simulink subsystem "Communication"  (R2022b)
settings: Solver=VariableStepAuto  StartTime=0.0  StopTime=10.0  RelTol=1e-3
values from neighbouring files (symbols this model uses):
  PWMclock = 100000000    [SimDefaultParam.mat]
undefined symbols (not defined in the file or in its folder): Fi, ODR, samplerate_serial, samplerate_udp, Wi
libraries: arduinowifilib x3, svdutilitieslib x2, simulink x1, arduinosensorlib x1
settings Model: Creator=ReiterTo  LastModifiedBy=ReiterTo

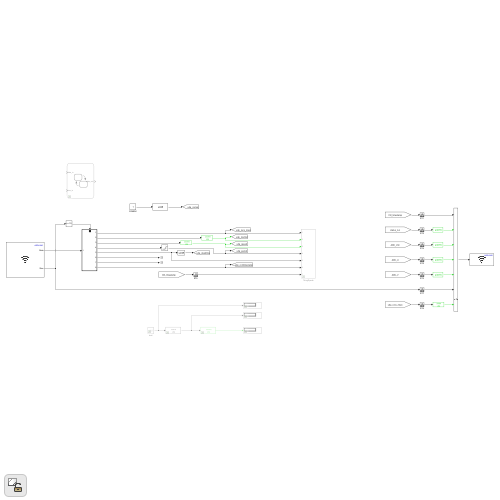
[thumbnail: Simulink's stored preview of the top-level diagram]
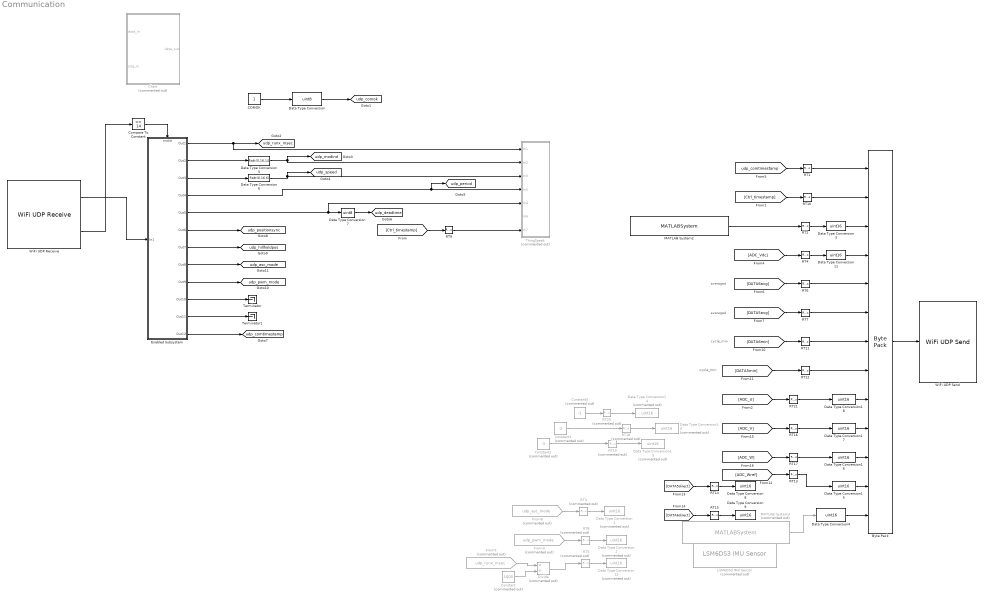
== system Communication ==
  note: averaged
  note: averaged
  note: cycle_min
  note: cycle_min
  Byte Pack : svdutilitieslib/Byte Pack  maskPackedDataType=uint16  datatypes={'uint32','uint32','uint16','uint16','uint16','uint16','uint16','uint16','uint16','uint16','uint16','uint16','uint16'}  byteAlign=2  blockPlatform=arduinoert
  COMOK : Constant  SampleTime=samplerate_serial
  Chart : Stateflow chart  Commented=on  TreatAsAtomicUnit=on
  Compare To Constant : simulink/Logic and Bit Operations/Compare To Constant  relop===  const=14  OutDataTypeStr=uint8
  Constant : Constant  Commented=on  Value=1000  OutDataTypeStr=uint16  SampleTime=samplerate_udp
  Constant1 : Constant  Commented=on  Value=-2  OutDataTypeStr=int16  SampleTime=samplerate_udp
  Constant2 : Constant  Commented=on  Value=-3  OutDataTypeStr=int16  SampleTime=samplerate_udp
  Constant3 : Constant  Commented=on  Value=-1  OutDataTypeStr=int16  SampleTime=samplerate_udp
  Data Type Conversion : DataTypeConversion  OutDataTypeStr=uint8  RndMeth=Simplest  SaturateOnIntegerOverflow=off
  Data Type Conversion1 : DataTypeConversion  Commented=on  OutDataTypeStr=uint16  RndMeth=Simplest  SaturateOnIntegerOverflow=off
  Data Type Conversion10 : DataTypeConversion  Commented=on  OutDataTypeStr=uint16  ConvertRealWorld=Stored Integer (SI)  RndMeth=Simplest  SaturateOnIntegerOverflow=off
  Data Type Conversion{3..4,8..9,11} (5 alike) : DataTypeConversion  OutDataTypeStr=uint16  RndMeth=Simplest  SaturateOnIntegerOverflow=off
  Data Type Conversion12 : DataTypeConversion  Commented=on  OutDataTypeStr=uint16  RndMeth=Simplest  SaturateOnIntegerOverflow=off
  Data Type Conversion13 : DataTypeConversion  Commented=on  OutDataTypeStr=uint16  ConvertRealWorld=Stored Integer (SI)  RndMeth=Simplest  SaturateOnIntegerOverflow=off
  Data Type Conversion14 : DataTypeConversion  Commented=on  OutDataTypeStr=uint16  ConvertRealWorld=Stored Integer (SI)  RndMeth=Simplest  SaturateOnIntegerOverflow=off
  Data Type Conversion{15..18} (4 alike) : DataTypeConversion  OutDataTypeStr=uint16  ConvertRealWorld=Stored Integer (SI)  RndMeth=Simplest  SaturateOnIntegerOverflow=off
  Data Type Conversion2 : DataTypeConversion  Commented=on  OutDataTypeStr=uint16  RndMeth=Simplest  SaturateOnIntegerOverflow=off
  Data Type Conversion5 : DataTypeConversion  OutDataTypeStr=fixdt(0,16,14)  ConvertRealWorld=Stored Integer (SI)  RndMeth=Simplest  SaturateOnIntegerOverflow=off  LockScale=on
  Data Type Conversion6 : DataTypeConversion  OutDataTypeStr=fixdt(0,16,6)  ConvertRealWorld=Stored Integer (SI)  RndMeth=Simplest  SaturateOnIntegerOverflow=off  LockScale=on
  Data Type Conversion7 : DataTypeConversion  OutDataTypeStr=uint8  RndMeth=Simplest  SaturateOnIntegerOverflow=off
  Divide : Product  Commented=on  Inputs=*/  OutDataTypeStr=uint32  RndMeth=Simplest
  Enabled Subsystem : Subsystem  TreatAsAtomicUnit=on
  From3 : From  Commented=on  GotoTag=udp_pwm_mode  TagVisibility=global
  From8 : From  Commented=on  GotoTag=udp_asc_mode  TagVisibility=global
  From9 : From  Commented=on  GotoTag=udp_runx_msec  TagVisibility=global
  LSM6DS3 IMU Sensor : arduinosensorlib/LSM6DS3 IMU Sensor  Commented=on  I2CAddress=0x6A  IsActiveAcceleration=off  IsActiveAngularRate=off  IsActiveTemperature=on  IsActiveStatus=off  IsActiveTimeStamp=off  spf=1  SampleTime=1  QueueSizeFactor=1  AccelerometerRange=+/- 2g  AccelerometerODR=12.5 Hz  SelectAnalogBW=off  AccelLPF1BW=400 Hz  AccelSelectCompositeFilter=No filter  AccelLPF2BW=ODR/50  AccelHPFBW=ODR/100  GyroscopeRange=250 dps  GyroscopeODR=12.5 Hz  SelectGyroscopeHPF=off  GyroHPFBW=0.0081 Hz
  MATLAB System2 : MATLABSystem  System=invPWM_Status
      mask Type: invPWM_Status
      mask Display:
      | disp('Inverter PWM Arduino Nano 33 IoT');
      | port_label('output',1,'pwm_run');
  MATLAB System3 : MATLABSystem  Commented=on  System=invSPI
      mask Type: invSPI
      mask Display:
      | disp('Inverter SPI Arduino Nano 33 IoT');
      | port_label('output',1,'DCL_RAW');
  RT{1..2,4,6..7,10..17,21} (14 alike) : RateTransition  Integrity=off  Deterministic=off  OutPortSampleTime=samplerate_udp
  RT{3,5,8,18..20} (6 alike) : RateTransition  Commented=on  Integrity=off  Deterministic=off  OutPortSampleTime=samplerate_udp
  RT9 : RateTransition  Integrity=off  Deterministic=off  OutPortSampleTime=samplerate_serial
  Terminator : Terminator
  Terminator1 : Terminator
  ThingSpeak : Subsystem  Commented=on
  WiFi UDP Receive : arduinowifilib/WiFi UDP Receive  localport=50000  DataType=uint16  DataLength=14  SampleTime_=samplerate_udp  wifiUDPIndex=0  blockPlatform=ARDUINO  isARMArch=true
  WiFi UDP Send : arduinowifilib/WiFi UDP Send  remoteIPOctetString=255.255.255.255  remoteport=60000  localport=50000  remoteipoctet1=255  remoteipoctet2=255  remoteipoctet3=255  remoteipoctet4=255  wifiUDPIndex=0  blockPlatform=ARDUINO  isARMArch=true
  tag scope: udp_asc_mode=global, udp_comok=global, udp_comtimestamp=global, udp_deadtime=global, udp_hillholdpos=global, udp_modind=global, udp_period=global, udp_positionsync=global, udp_pwm_mode=global, udp_runx_msec=global, udp_speed=global
  wires:
  Data Type Conversion/1 -> [udp_comok]
  [Ctrl_timestamp] -> RT9/1
  COMOK/1 -> Data Type Conversion/1
  RT2/1 -> Data Type Conversion3/1
  MATLAB System2/1 -> RT2/1
  RT1/1 -> Byte Pack/1
  Byte Pack/1 -> WiFi UDP Send/1
  Data Type Conversion6/1 -> ThingSpeak/3(In3), [udp_speed]
  Data Type Conversion7/1 -> [udp_deadtime]
  Enabled Subsystem/4(Out4) -> [udp_period], ThingSpeak/4(In5)
  [ADC_Vdc] -> RT4/1
  RT4/1 -> Data Type Conversion11/1
  From9/1 -> Divide/1
  RT5/1 -> Data Type Conversion12/1
  RT9/1 -> ThingSpeak/7(In7)
  RT3/1 -> Data Type Conversion1/1
  Data Type Conversion5/1 -> [udp_modind], ThingSpeak/2(In2)
  Enabled Subsystem/1(Out1) -> ThingSpeak/1(In1), [udp_runx_msec]
  Enabled Subsystem/5(Out5) -> Data Type Conversion7/1, ThingSpeak/5(In4)
  WiFi UDP Receive/1 -> Enabled Subsystem/1(In1)
  Enabled Subsystem/2(Out2) -> Data Type Conversion5/1
  Enabled Subsystem/3(Out3) -> Data Type Conversion6/1
  Enabled Subsystem/6(Out6) -> [udp_positionsync]
  Enabled Subsystem/7(Out7) -> [udp_hillholdpos]
  [DATA5avg] -> RT7/1
  [DATA6avg] -> RT6/1
  RT8/1 -> Data Type Conversion2/1
  WiFi UDP Receive/2 -> Compare To Constant/1
  Compare To Constant/1 -> Enabled Subsystem/Enable
  From3/1 -> RT8/1
  From8/1 -> RT3/1
  Enabled Subsystem/8(Out8) -> [udp_asc_mode]
  Enabled Subsystem/9(Out9) -> [udp_pwm_mode]
  Enabled Subsystem/10(Out10) -> Terminator/1
  Enabled Subsystem/11(Out11) -> Terminator1/1
  Divide/1 -> RT5/1
  Constant/1 -> Divide/2
  Enabled Subsystem/12(Out12) -> [udp_comtimestamp]
  [udp_comtimestamp] -> RT1/1
  [Ctrl_timestamp] -> RT10/1
  RT10/1 -> Byte Pack/2
  [DATA6min] -> RT11/1
  [DATA5min] -> RT12/1
  Data Type Conversion3/1 -> Byte Pack/3
  Data Type Conversion11/1 -> Byte Pack/4
  RT6/1 -> Byte Pack/5
  RT7/1 -> Byte Pack/6
  RT11/1 -> Byte Pack/7
  RT12/1 -> Byte Pack/8
  [DATA5direct] -> RT14/1
  RT14/1 -> Data Type Conversion8/1
  RT15/1 -> Data Type Conversion9/1
  [DATA6direct] -> RT15/1
  [ADC_V] -> RT16/1
  [ADC_W] -> RT17/1
  RT18/1 -> Data Type Conversion10/1
  [ADC_Wref] -> RT13/1
  RT13/1 -> Data Type Conversion15/1
  Data Type Conversion4/1 -> Byte Pack/13
  MATLAB System3/1 -> Data Type Conversion4/1
  Constant1/1 -> RT18/1
  RT19/1 -> Data Type Conversion13/1
  Constant2/1 -> RT19/1
  RT20/1 -> Data Type Conversion14/1
  Constant3/1 -> RT20/1
  Data Type Conversion15/1 -> Byte Pack/12
  Data Type Conversion16/1 -> Byte Pack/11
  Data Type Conversion17/1 -> Byte Pack/10
  Data Type Conversion18/1 -> Byte Pack/9
  RT17/1 -> Data Type Conversion16/1
  RT16/1 -> Data Type Conversion17/1
  RT21/1 -> Data Type Conversion18/1
  [ADC_U] -> RT21/1

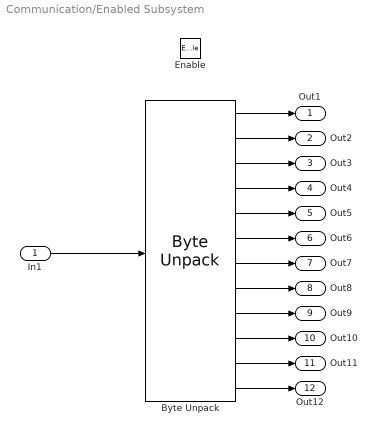
== system Communication/Enabled Subsystem ==
  In1 : Inport
  Enable : EnablePort
  Byte Unpack : svdutilitieslib/Byte Unpack  dimensions={[1],[1],[1],[1],[1],[1],[1],[1],[1],[1],[1],[1]}  datatypes={'uint32','uint16','uint16','uint16','uint16','uint16','uint16','uint16','uint16','uint16','uint16','uint32'}  byteAlign=2  blockPlatform=arduinoert
  Out1 : Outport
  Out2 : Outport  Port=2
  Out3 : Outport  Port=3
  Out4 : Outport  Port=4
  Out5 : Outport  Port=5
  Out6 : Outport  Port=6
  Out7 : Outport  Port=7
  Out8 : Outport  Port=8
  Out9 : Outport  Port=9
  Out10 : Outport  Port=10
  Out11 : Outport  Port=11
  Out12 : Outport  Port=12
  wires:
  Byte Unpack/12 -> Out12/1
  Byte Unpack/11 -> Out11/1
  Byte Unpack/10 -> Out10/1
  Byte Unpack/9 -> Out9/1
  Byte Unpack/8 -> Out8/1
  Byte Unpack/7 -> Out7/1
  Byte Unpack/6 -> Out6/1
  Byte Unpack/5 -> Out5/1
  Byte Unpack/4 -> Out4/1
  Byte Unpack/3 -> Out3/1
  Byte Unpack/2 -> Out2/1
  Byte Unpack/1 -> Out1/1
  In1/1 -> Byte Unpack/1

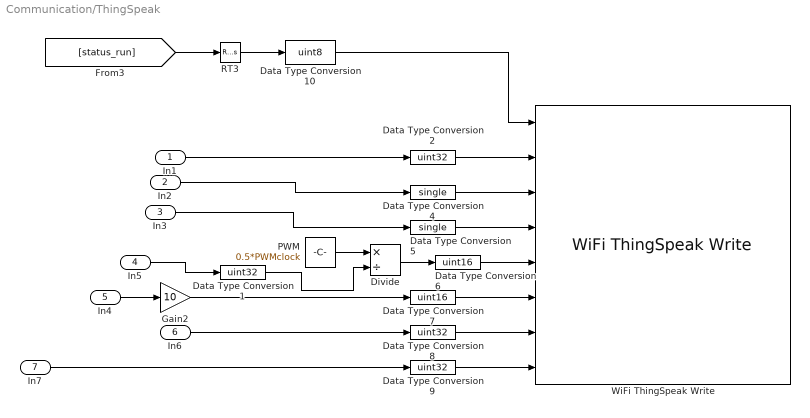
== system Communication/ThingSpeak ==
  In1 : Inport
  In2 : Inport  Port=2
  In3 : Inport  Port=3
  In5 : Inport  Port=4
  In4 : Inport  Port=5
  In6 : Inport  Port=6
  In7 : Inport  Port=7
  Data Type Conversion{1..2,8..9} (4 alike) : DataTypeConversion  OutDataTypeStr=uint32  SaturateOnIntegerOverflow=off  RndMeth=Floor
  Data Type Conversion10 : DataTypeConversion  OutDataTypeStr=uint8  SaturateOnIntegerOverflow=off  RndMeth=Floor
  Data Type Conversion4 : DataTypeConversion  OutDataTypeStr=single  SaturateOnIntegerOverflow=off  RndMeth=Floor
  Data Type Conversion5 : DataTypeConversion  OutDataTypeStr=single  SaturateOnIntegerOverflow=off  RndMeth=Floor
  Data Type Conversion6 : DataTypeConversion  OutDataTypeStr=uint16  SaturateOnIntegerOverflow=off  RndMeth=Floor
  Data Type Conversion7 : DataTypeConversion  OutDataTypeStr=uint16  SaturateOnIntegerOverflow=off  RndMeth=Floor
  Divide : Product  Inputs=*/  RndMeth=Simplest
  Gain2 : Gain  Gain=10  OutDataTypeStr=uint16  RndMeth=Simplest
  PWM : Constant  Value=0.5*PWMclock  OutDataTypeStr=uint32  SampleTime=samplerate_serial
  RT3 : RateTransition  Integrity=off  Deterministic=off  OutPortSampleTime=samplerate_serial
  WiFi ThingSpeak Write : arduinowifilib/WiFi ThingSpeak Write  ChannelID_=2477243  WriteAPIKey_=Z6BZPM8LP3Z3KJLJ  FieldsToWrite=[1 2 3 4 5 6 7 8]  UpdateInterval_=15  PrintDiagnosticMessages_=off  LocationEnabled=off  LocationSource=Input port  blockPlatform=arduino  Interfacetype_=Wi-Fi  UpdateURL=0  StatusMessage=0  StatusEnabled=on  StatusSource=<empty>
  wires:
  Gain2/1 -> Data Type Conversion7/1
  In3/1 -> Data Type Conversion5/1
  In2/1 -> Data Type Conversion4/1
  In5/1 -> Data Type Conversion1/1
  In7/1 -> Data Type Conversion9/1
  In4/1 -> Gain2/1
  In1/1 -> Data Type Conversion2/1
  Data Type Conversion7/1 -> WiFi ThingSpeak Write/6
  RT3/1 -> Data Type Conversion10/1
  [status_run] -> RT3/1
  Data Type Conversion2/1 -> WiFi ThingSpeak Write/2
  Divide/1 -> Data Type Conversion6/1
  Data Type Conversion6/1 -> WiFi ThingSpeak Write/5
  Data Type Conversion8/1 -> WiFi ThingSpeak Write/7
  Data Type Conversion10/1 -> WiFi ThingSpeak Write/1
  Data Type Conversion9/1 -> WiFi ThingSpeak Write/8
  PWM/1 -> Divide/1
  Data Type Conversion1/1 -> Divide/2
  Data Type Conversion5/1 -> WiFi ThingSpeak Write/4
  Data Type Conversion4/1 -> WiFi ThingSpeak Write/3
  In6/1 -> Data Type Conversion8/1

== stateflow chart Communication/Chart ==
  state NewData
    en: data_out = data_in;
  (default) -> NewData
  (junction 17) -> NewData
  NewData -> (junction 17) : [size_in ~= 0]
  data: data_in input uint16 size=10; data_out output uint16 size=10; size_in input uint16 size=1
